simulink model "SSB"  (R2020b)
settings: Solver=VariableStepAuto  StartTime=0.0  StopTime=10.0  RelTol=1e-3
libraries: dsparch4 x2
settings Model: Creator=htn  LastModifiedBy=htn

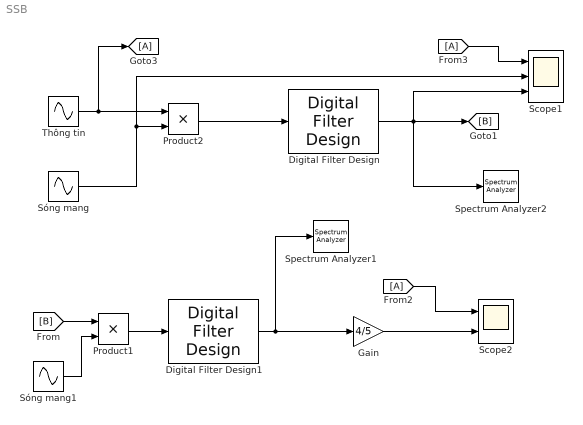
== system SSB ==
  Digital Filter Design : dsparch4/Digital Filter Design  mwdsp_browser_bugfix_var=off
  Digital Filter Design1 : dsparch4/Digital Filter Design  mwdsp_browser_bugfix_var=off
  Gain : Gain  Gain=4/5
  Product1 : Product
  Product2 : Product
  Scope1 : Scope  NumInputPorts=3
  Scope2 : Scope  NumInputPorts=2
  Spectrum Analyzer1 : SpectrumAnalyzer
  Spectrum Analyzer2 : SpectrumAnalyzer
  Sóng mang : Sin  Amplitude=5  Frequency=2*pi*5000  SampleTime=1/50000
  Sóng mang1 : Sin  Frequency=2*pi*5000  SampleTime=1/50000
  Thông tin : Sin  Frequency=2*pi*1000  SampleTime=1/50000
  wires:
  Thông tin/1 -> Product2/1, [A]
  Sóng mang/1 -> Product2/2, Scope1/2
  Product2/1 -> Digital Filter Design/1
  [A] -> Scope1/1
  Digital Filter Design/1 -> Spectrum Analyzer2/1, [B], Scope1/3
  Gain/1 -> Scope2/2
  Digital Filter Design1/1 -> Gain/1, Spectrum Analyzer1/1
  [A] -> Scope2/1
  [B] -> Product1/1
  Sóng mang1/1 -> Product1/2
  Product1/1 -> Digital Filter Design1/1
